simulink model "HodkinHuxley_ecg"  (Simulink 6.6)
settings: Solver=ode45  StartTime=0.0  StopTime=50.0  RelTol=1e-3
libraries: simulink x1
settings Model: Creator=MXKana  LastModifiedBy=mxkana

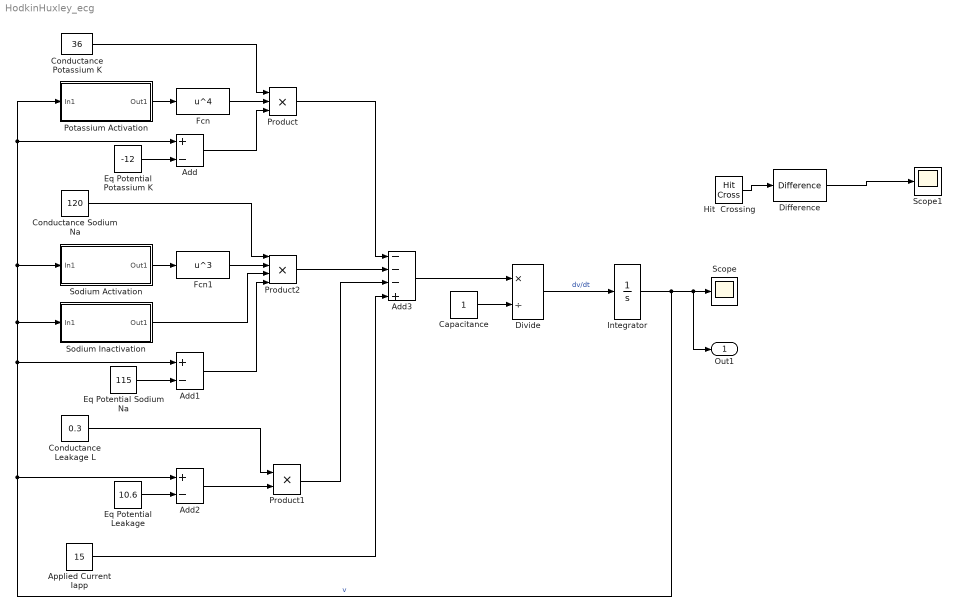
== system HodkinHuxley_ecg ==
  Add : Sum  Inputs=+-  OutScaling=2^-10
  Add1 : Sum  Inputs=+-  OutScaling=2^-10
  Add2 : Sum  Inputs=+-  OutScaling=2^-10
  Add3 : Sum  Inputs=---+  OutScaling=2^-10
  Applied Current Iapp : Constant  Value=15
  Capacitance : Constant
  Conductance Leakage L : Constant  Value=0.3
  Conductance Potassium K : Constant  Value=36
  Conductance Sodium Na : Constant  Value=120
  Difference : simulink/Discrete/Difference  SystemSampleTime=-1  ICPrevInput=2  OutDataType=sfix(16)  OutScaling=2^-10  DoSatur=off
  Divide : Product  Inputs=*/  OutScaling=2^-10
  Eq Potential Leakage : Constant  Value=10.6
  Eq Potential Potassium K : Constant  Value=-12
  Eq Potential Sodium Na : Constant  Value=115
  Fcn : Fcn  Expr=u^4
  Fcn1 : Fcn  Expr=u^3
  Hit  Crossing : HitCross  HitCrossingOffset=60  HitCrossingDirection=rising
  Integrator : Integrator
  Potassium Activation : Subsystem
  Product : Product  Inputs=3  RndMeth=Zero
  Product1 : Product  RndMeth=Zero
  Product2 : Product  Inputs=4  RndMeth=Zero
  Scope : Scope
      settings: YMin=-20  YMax=120
  Scope1 : Scope
      settings: YMin=-20  YMax=120
  Sodium Activation : Subsystem
  Sodium Inactivation : Subsystem
  Out1 : Outport
  wires:
  Capacitance/1 -> Divide/2
  Conductance Potassium K/1 -> Product/1
  Potassium Activation/1(Out1) -> Fcn/1
  Fcn/1 -> Product/2
  Conductance Sodium Na/1 -> Product2/1
  Sodium Activation/1(Out1) -> Fcn1/1
  Fcn1/1 -> Product2/2
  Sodium Inactivation/1(Out1) -> Product2/3
  Eq Potential Potassium K/1 -> Add/2
  Add/1 -> Product/3
  Eq Potential Sodium Na/1 -> Add1/2
  Add1/1 -> Product2/4
  Eq Potential Leakage/1 -> Add2/2
  Add2/1 -> Product1/2
  Conductance Leakage L/1 -> Product1/1
  Product/1 -> Add3/1
  Product2/1 -> Add3/2
  Product1/1 -> Add3/3
  Applied Current Iapp/1 -> Add3/4
  Add3/1 -> Divide/1
  Divide/1 -> Integrator/1  "dv/dt"
  Integrator/1 -> Add/1, Potassium Activation/1(In1), Sodium Activation/1(In1), Sodium Inactivation/1(In1), Add1/1, Add2/1, Scope/1, Out1/1  "v"
  Hit  Crossing/1 -> Difference/1
  Difference/1 -> Scope1/1

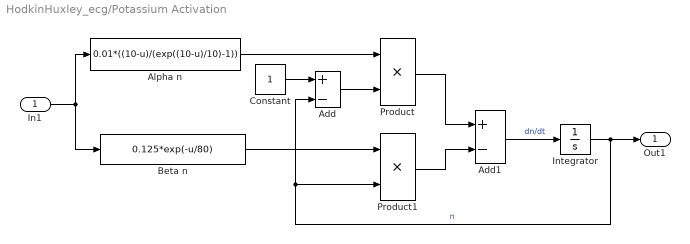
== system HodkinHuxley_ecg/Potassium Activation ==
  In1 : Inport
  Add : Sum  Inputs=+-  OutScaling=2^-10
  Add1 : Sum  Inputs=+-  OutScaling=2^-10
  Alpha n : Fcn  Expr=0.01*((10-u)/(exp((10-u)/10)-1))
  Beta n : Fcn  Expr=0.125*exp(-u/80)
  Constant : Constant
  Integrator : Integrator
  Product : Product  RndMeth=Zero
  Product1 : Product  RndMeth=Zero
  Out1 : Outport
  wires:
  In1/1 -> Alpha n/1, Beta n/1
  Constant/1 -> Add/1
  Alpha n/1 -> Product/1
  Add/1 -> Product/2
  Beta n/1 -> Product1/1
  Product/1 -> Add1/1
  Product1/1 -> Add1/2
  Add1/1 -> Integrator/1  "dn/dt"
  Integrator/1 -> Add/2, Product1/2, Out1/1  "n"

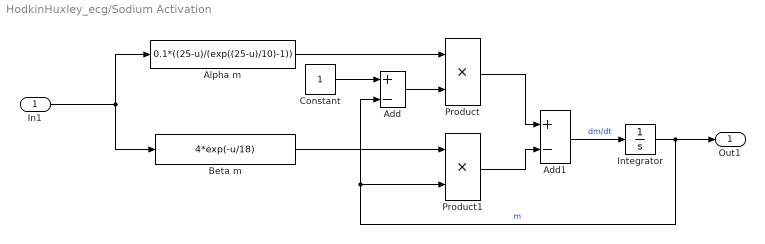
== system HodkinHuxley_ecg/Sodium Activation ==
  In1 : Inport
  Add : Sum  Inputs=+-  OutScaling=2^-10
  Add1 : Sum  Inputs=+-  OutScaling=2^-10
  Alpha m : Fcn  Expr=0.1*((25-u)/(exp((25-u)/10)-1))
  Beta m : Fcn  Expr=4*exp(-u/18)
  Constant : Constant
  Integrator : Integrator
  Product : Product  RndMeth=Zero
  Product1 : Product  RndMeth=Zero
  Out1 : Outport
  wires:
  In1/1 -> Alpha m/1, Beta m/1
  Constant/1 -> Add/1
  Alpha m/1 -> Product/1
  Add/1 -> Product/2
  Beta m/1 -> Product1/1
  Product/1 -> Add1/1
  Product1/1 -> Add1/2
  Add1/1 -> Integrator/1  "dm/dt"
  Integrator/1 -> Add/2, Product1/2, Out1/1  "m"

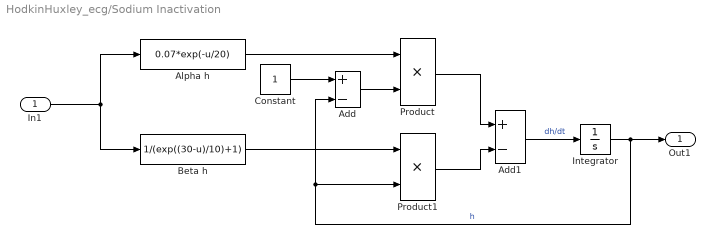
== system HodkinHuxley_ecg/Sodium Inactivation ==
  In1 : Inport
  Add : Sum  Inputs=+-  OutScaling=2^-10
  Add1 : Sum  Inputs=+-  OutScaling=2^-10
  Alpha h : Fcn  Expr=0.07*exp(-u/20)
  Beta h : Fcn  Expr=1/(exp((30-u)/10)+1)
  Constant : Constant
  Integrator : Integrator
  Product : Product  RndMeth=Zero
  Product1 : Product  RndMeth=Zero
  Out1 : Outport
  wires:
  In1/1 -> Alpha h/1, Beta h/1
  Constant/1 -> Add/1
  Alpha h/1 -> Product/1
  Add/1 -> Product/2
  Beta h/1 -> Product1/1
  Product/1 -> Add1/1
  Product1/1 -> Add1/2
  Add1/1 -> Integrator/1  "dh/dt"
  Integrator/1 -> Add/2, Product1/2, Out1/1  "h"
